simulink model "SimpleCam_UCS"  (R2025b)
settings: Solver=FixedStepDiscrete  StartTime=0.0  StopTime=tspan  FixedStep=dt_sim  RelTol=1e-3
model workspace (MAT data in the model file):
  socvcb = containers.Map
  socvcb.serialization.keys = {}
  socvcb.serialization.values = {}
  socvcb.serialization.uniformity = 0
  socvcb.serialization.keyType = 'double'
  socvcb.serialization.valueType = 'any'
undefined symbols (not defined in the file): dt_sample, exactDistance_KP, exactPhi_KP, exactTheta_KP, gate1_Pose, M_UCSToWorld, M_WorldToUCS, rel_CamPose_L_UCS, rel_CamPose_R_UCS, Sim3dSensor
libraries: sim3dlib x3, sim3dcameralib x2, visionsinks x2
settings Model: Creator=Liam  LastModifiedBy=Liam

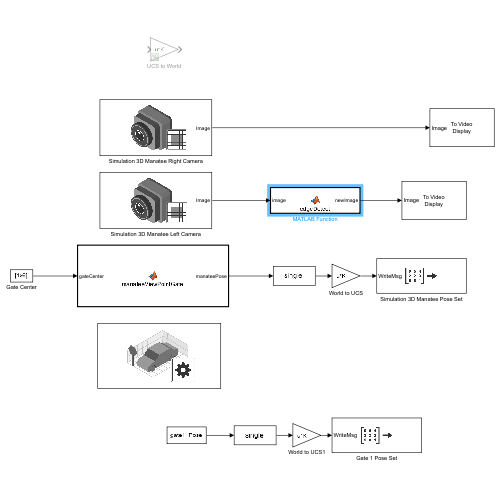
[thumbnail: Simulink's stored preview of the top-level diagram]
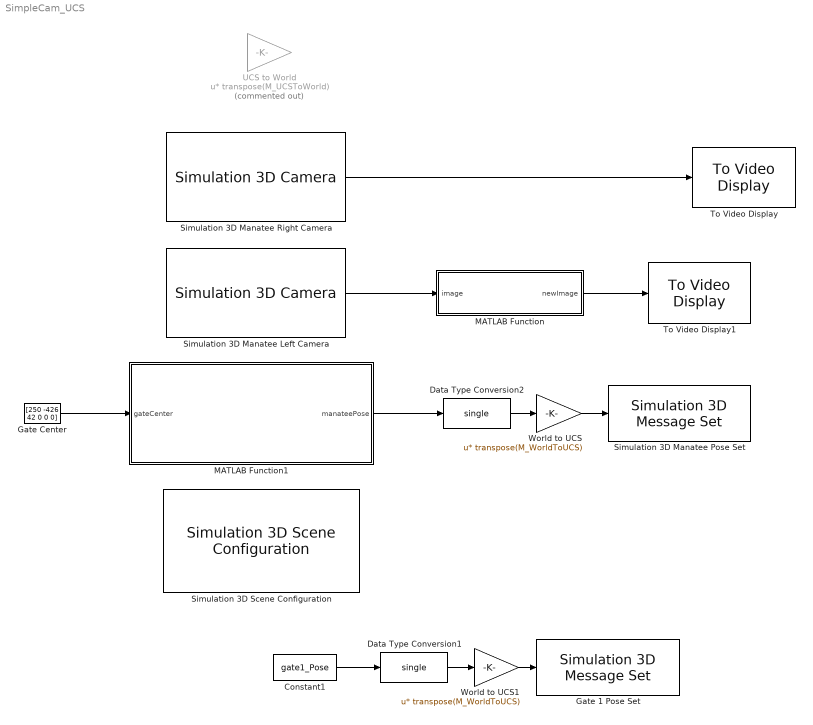
== system SimpleCam_UCS ==
  Constant1 : Constant  Value=gate1_Pose  VectorParams1D=off  OutDataTypeStr=single
  Data Type Conversion1 : DataTypeConversion  OutDataTypeStr=single  SaturateOnIntegerOverflow=off  RndMeth=Floor
  Data Type Conversion2 : DataTypeConversion  OutDataTypeStr=single  SaturateOnIntegerOverflow=off  RndMeth=Floor
  Gate 1 Pose Set : sim3dlib/Simulation 3D Message Set  Priority=-1  SigName=Gate1PoseSet  Ts=-1  aMode=0
      settings: LibrarySourceBlock=aerolibsim3d/Simulation 3D Message Set
  Gate Center : Constant  Value=[250 -426 42 0 0 0]  VectorParams1D=off  OutDataTypeStr=single  SampleTime=-1
  MATLAB Function : MATLAB Function  TreatAsAtomicUnit=on
  MATLAB Function1 : MATLAB Function  TreatAsAtomicUnit=on
  Simulation 3D Manatee Left Camera : sim3dcameralib/Simulation 3D Camera  Priority=1  sensorTag=Sim3dSensor�  sensorId=1  sensorName=Sim3dSensor�  vehTagList={'Scene Origin'}  vehTag=Scene Origin  CoordinateSystem=Default  mountLoc=Origin  offsetFlag=on  tmountOffset=rel_CamPose_L_UCS(1:3) / 100  extTmount=off  rmountOffset=rel_CamPose_L_UCS(4:6)  extRmount=off  FocalLength=[2.97 / 0.0028, 2.97 / 0.0028]  OpticalCenter=[960, 540]  ImageSize=[1080, 1920]  RadialDistortion=[0.33 0.16]  TangentialDistortion=[0 0]  SensorSkew=0  VisualizeFieldOfView=off  FieldOfViewRange=61  DepthOutportEnabled=off  SemanticOutportEnabled=off  TransformOutportEnabled=off  SampleTime=dt_sample  mountPoint=[0.4 -0.125 0.15]  mountOrientation=[0 0 0]  aMode=5  ID=1
      settings: LibrarySourceBlock=sl3dlib/Simulation 3D/Sensors/Simulation 3D Camera
  Simulation 3D Manatee Pose Set : sim3dlib/Simulation 3D Message Set  Priority=-1  SigName=ManateePoseSet  Ts=dt_sample  aMode=0
      settings: LibrarySourceBlock=aerolibsim3d/Simulation 3D Message Set
  Simulation 3D Manatee Right Camera : sim3dcameralib/Simulation 3D Camera  Priority=1  sensorTag=Sim3dSensor�  sensorId=2  sensorName=Sim3dSensor�  vehTagList={'Scene Origin'}  vehTag=Scene Origin  CoordinateSystem=Default  mountLoc=Origin  offsetFlag=on  tmountOffset=rel_CamPose_R_UCS(1:3) / 100  extTmount=off  rmountOffset=rel_CamPose_R_UCS(4:6)  extRmount=off  FocalLength=[2.97 / 0.0028, 2.97 / 0.0028]  OpticalCenter=[960, 540]  ImageSize=[1080, 1920]  RadialDistortion=[0.33 0.16]  TangentialDistortion=[0 0]  SensorSkew=0  VisualizeFieldOfView=off  FieldOfViewRange=61  DepthOutportEnabled=off  SemanticOutportEnabled=off  TransformOutportEnabled=off  SampleTime=dt_sample  mountPoint=[0.4 0.125 0.15]  mountOrientation=[0 0 0]  aMode=5  ID=2
      settings: LibrarySourceBlock=sl3dlib/Simulation 3D/Sensors/Simulation 3D Camera
  Simulation 3D Scene Configuration : sim3dlib/Simulation 3D Scene Configuration  Priority=0  ProjectFormat=Unreal Executable  SceneDesc=Straight road  ProjectName=C:\Users\Liam\OneDrive\Documents\GitHub\SimulinkPlant\DROP UCS PACKAGED BUILD HERE\EllingtonPoolSim.exe  ScenePath=/Game/Prop_Test_Level  UEProjPath=C:\Users\Liam\OneDrive\Documents\GitHub\Vision_Sim\Unreal\UnrealProjects\SimulinkCoSimulation\EllingtonPoolSim\EllingtonPoolSim.uproject  EnableOpenDRIVE=off  vehTagList={'Custom';'Scene Origin'}  vehTag=Scene Origin  AttachedCameraRelativeTranslation=[0 0 0]  FreeCameraDefaultInitialTranslation=[-6, 0, 2]  AttachedCameraRelativeRotation=[0 0 0]  FreeCameraDefaultInitialRotation=[0, -15, 0]  ViewpointName=Custom  FreeCameraInitialTranslation=[0, 0, 0]  ViewpointTranslation=[0 0 0]  FreeCameraInitialRotation=[0, 0, 0]  ViewpointRotation=[0 0 0]  OpVisEn=off  Ts=dt_sample  EnableWindow=on  EnableRemoteAccess=off  EnableWeather=off  SunAzimuth=90  SunAltitude=40.0  EnableGeospatialSun=off  Latitude=0  Longitude=0  Date=2023-01-01  Time=10:30:00  GeoTimeZone=-5.0  SunDaylightSaving=off  wind=1  clouds=10  EnableVolumetricClouds=off  CloudCoverage=0  CloudAltitude=6  fog=0  rain=0  RaindropsEffect=off  SnowDensity=0  EnableGeospatial=off  TilesetSource=Earth terrain  UseTrueOrigin=off  OriginHeight=200  OriginLatitude=40.744652  OriginLongitude=-73.988864  MapStyle=Aerial  AdditionalAssetIDs=[]  UseAdvancedSunSky=off  SolarTime=11  TimeZone=-5  Day=21  Month=9  Year=2022  UseDaylightSavingTime=on  DSTStartDay=10  DSTStartMonth=3  DSTEndDay=3  DSTEndMonth=11  DSTSwitchHour=2  sensorTag=MainCamera1  sensorId=1  sensorName=MainCamera1  mountLoc=Origin  offsetFlag=off  tmountOffset=[0, 0, 0]  rmountOffset=[0, 0, 0]  HorizontalResolution=1280  VerticalResolution=720  HorizontalFOV=60  mountPoint=[0 0 0]  mountOrientation=[0 0 0]  aMode=3  ID=1  GeoTrigger=Inactive  ViewNameList={'Custom'}  ViewTranslationList={'[0 0 0]'}  ViewRotationList={'[0 0 0]'}
      settings: LibrarySourceBlock=drivingsim3d/Simulation 3D Scene Configuration
  To Video Display : visionsinks/To Video Display  windowSizeMode=Normal  openAtMdlStart=on  fullScreen=off  videoWindowX=536805376  videoWindowY=536805376  saveWindowSize=off  videoWindowWidth=1920  videoWindowHeight=1080  inputColorFormat=RGB  inputType=Obsolete  imagePorts=One multidimensional signal  OutputDevice=On-screen video monitor  dataOrg=Column-major  isWindowOpen=off
  To Video Display1 : visionsinks/To Video Display  windowSizeMode=Normal  openAtMdlStart=on  fullScreen=off  videoWindowX=536805376  videoWindowY=536805376  saveWindowSize=off  videoWindowWidth=1920  videoWindowHeight=1080  inputColorFormat=RGB  inputType=Obsolete  imagePorts=One multidimensional signal  OutputDevice=On-screen video monitor  dataOrg=Column-major  isWindowOpen=off
  UCS to World : Gain  Commented=on  Gain=transpose(M_UCSToWorld)  Multiplication=Matrix(u*K)
  World to UCS : Gain  Gain=transpose(M_WorldToUCS)  Multiplication=Matrix(u*K)
  World to UCS1 : Gain  Gain=transpose(M_WorldToUCS)  Multiplication=Matrix(u*K)
  wires:
  Data Type Conversion2/1 -> World to UCS/1
  MATLAB Function1/1(manateePose) -> Data Type Conversion2/1
  Constant1/1 -> Data Type Conversion1/1
  Data Type Conversion1/1 -> World to UCS1/1
  World to UCS/1 -> Simulation 3D Manatee Pose Set/1
  World to UCS1/1 -> Gate 1 Pose Set/1
  Simulation 3D Manatee Left Camera/1 -> MATLAB Function/1(image)
  Gate Center/1 -> MATLAB Function1/1(gateCenter)
  Simulation 3D Manatee Right Camera/1 -> To Video Display/1
  MATLAB Function/1(newImage) -> To Video Display1/1

== matlab function SimpleCam_UCS/MATLAB Function1 ==
  settings: updateMethod=DISCRETE  sampleTime=dt_sample
  data: gateCenter input; manateePose output; exactDistance_KP parameter; exactPhi_KP parameter; exactTheta_KP parameter
function manateePose = manateeViewPointGate(gateCenter, exactDistance_KP, exactPhi_KP, exactTheta_KP)
x = exactDistance_KP * sin(exactTheta_KP) * cos(exactPhi_KP);
y = exactDistance_KP * sin(exactTheta_KP) * sin(exactPhi_KP);
z = exactDistance_KP * cos(exactTheta_KP);
manateeRoll = 0;
manateePitch = (pi / 2 - exactTheta_KP);
manateeYaw = exactPhi_KP - pi;
manateePose = [(gateCenter(1) + x) (gateCenter(2) + y) (gateCenter(3) + z) manateeRoll manateePitch  manateeYaw];

== matlab function SimpleCam_UCS/MATLAB Function ==
  data: image input; newImage output
function newImage = edgeDetect(image)

grayImage = im2gray(image);
%blueImage = image(:,:,1);

newImage = edge(grayImage, 'sobel');

%{
corners = detectHarrisFeatures(grayImage).Location;
squareSize = 5;
dimensions = size(corners);
for i = 1:dimensions(1)
    x = round(corners(i, 1));
    y = round(corners(i, 2));
    if x <= 1920 - squareSize && x > squareSize && y <= 1080 - squareSize && y > squareSize
        for xi = (x - squareSize):(x + squareSize)
            for yi = (y - squareSize):(y + squareSize)
                grayImage(yi,xi) = 255;
            end
        end
    end
end
%}



%newImage = grayImage;
